simulink library "courseFollow_cl"  (R2018b)
settings: Solver=VariableStepAuto  StartTime=0.0  StopTime=10.0  RelTol=1e-3
undefined symbols (not defined in the file or in its folder): a
libraries: schmehlTangentRotation_ul x1, angleBtw2DVecs_ul x1
settings Model: Creator=James Reed  LastModifiedBy=jldanie5

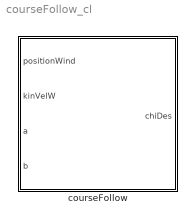
== system courseFollow_cl ==
  courseFollow : Subsystem

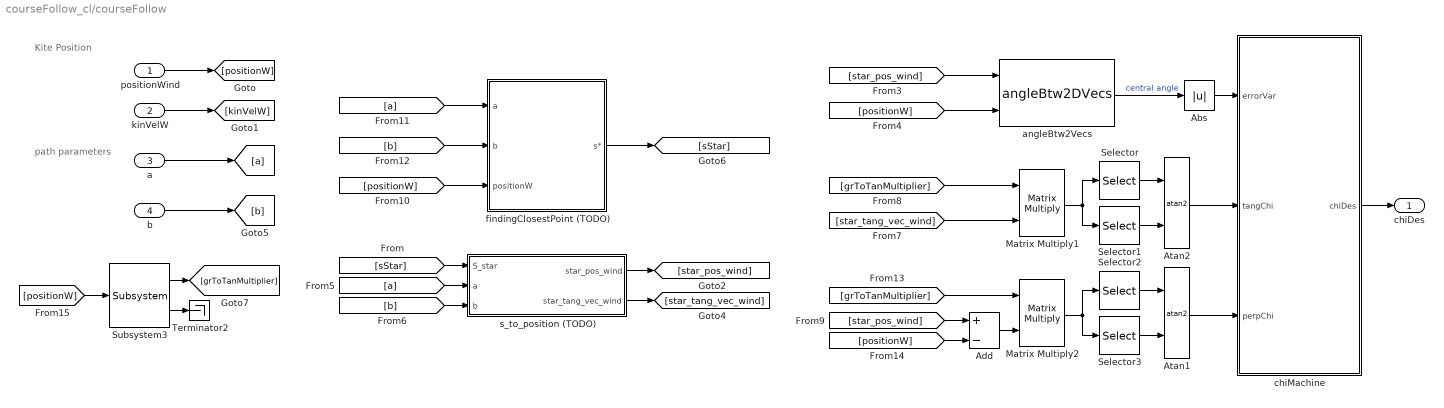
== system courseFollow_cl/courseFollow ==
  note: Kite Position
  note: path parameters
  "positionWind " : Inport
  kinVelW : Inport  Port=2
  a : Inport  Port=3
  "b " : Inport  Port=4
  Abs : Abs
  Add : Sum  Inputs=+-
  Atan1 : Trigonometry  Operator=atan2
  Atan2 : Trigonometry  Operator=atan2
  Matrix Multiply1 : Product  Multiplication=Matrix(*)
  Matrix Multiply2 : Product  Multiplication=Matrix(*)
  Selector : Selector  InputPortWidth=3  IndexOptions=Index vector (dialog)  Indices=2  OutputSizes=1
  Selector1 : Selector  InputPortWidth=3  IndexOptions=Index vector (dialog)  Indices=1  OutputSizes=1
  Selector2 : Selector  InputPortWidth=3  IndexOptions=Index vector (dialog)  Indices=2  OutputSizes=1
  Selector3 : Selector  InputPortWidth=3  IndexOptions=Index vector (dialog)  Indices=1  OutputSizes=1
  Subsystem3 : schmehlTangentRotation_ul/Subsystem  SystemSampleTime=-1
  Terminator2 : Terminator
  angleBtw2Vecs : angleBtw2DVecs_ul/angleBtw2DVecs  SystemSampleTime=-1
  chiMachine : Subsystem  mask{error_upper_lim=10*pi/180}
      mask prompts: error_upper_lim "Value of Error yielding 100% perpendicular"
  findingClosestPoint (TODO) : Subsystem
  s_to_position (TODO) : Subsystem
  "chiDes " : Outport
  wires:
  "positionWind "/1 -> [positionW]
  chiMachine/1("chiDes ") -> "chiDes "/1
  [positionW] -> findingClosestPoint (TODO)/3(positionW)
  a/1 -> [a]
  "b "/1 -> [b]
  [a] -> findingClosestPoint (TODO)/1(a)
  [b] -> findingClosestPoint (TODO)/2(b)
  findingClosestPoint (TODO)/1(s*) -> [sStar]
  [positionW] -> Subsystem3/1
  Subsystem3/2 -> Terminator2/1
  Subsystem3/1 -> [grToTanMultiplier]
  kinVelW/1 -> [kinVelW]
  [sStar] -> s_to_position (TODO)/1(S_star)
  s_to_position (TODO)/1(star_pos_wind) -> [star_pos_wind]
  [star_pos_wind] -> angleBtw2Vecs/1
  [positionW] -> angleBtw2Vecs/2
  angleBtw2Vecs/1 -> Abs/1  "central angle"
  Abs/1 -> chiMachine/1("errorVar ")
  [a] -> s_to_position (TODO)/2(a)
  [b] -> s_to_position (TODO)/3(b)
  s_to_position (TODO)/2(star_tang_vec_wind) -> [star_tang_vec_wind]
  Matrix Multiply1/1 -> Selector1/1, Selector/1
  [star_tang_vec_wind] -> Matrix Multiply1/2
  [grToTanMultiplier] -> Matrix Multiply1/1
  Selector/1 -> Atan2/1
  Selector1/1 -> Atan2/2
  Atan2/1 -> chiMachine/2(tangChi)
  [grToTanMultiplier] -> Matrix Multiply2/1
  Selector3/1 -> Atan1/2
  Matrix Multiply2/1 -> Selector3/1, Selector2/1
  Atan1/1 -> chiMachine/3("perpChi ")
  Selector2/1 -> Atan1/1
  Add/1 -> Matrix Multiply2/2
  [star_pos_wind] -> Add/1
  [positionW] -> Add/2

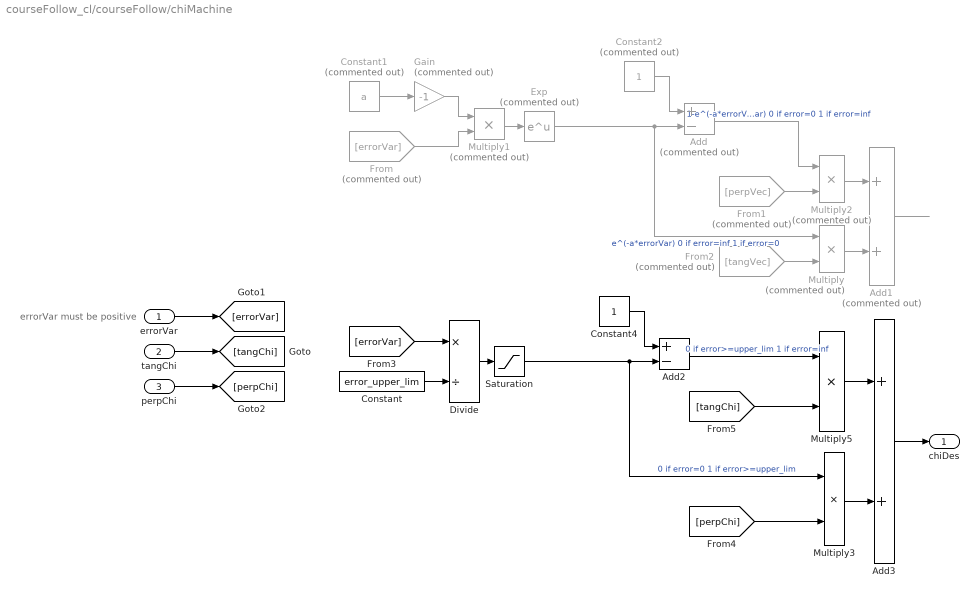
== system courseFollow_cl/courseFollow/chiMachine ==
  note: errorVar must be positive
  "errorVar " : Inport
  tangChi : Inport  Port=2
  "perpChi " : Inport  Port=3
  Add : Sum  Commented=on  Inputs=+-
  Add1 : Sum  Commented=on
  Add2 : Sum  Inputs=+-
  Add3 : Sum
  Constant : Constant  Value=error_upper_lim
  Constant1 : Constant  Commented=on  Value=a
  Constant2 : Constant  Commented=on
  Constant4 : Constant
  Divide : Product  Inputs=*/
  Exp : Math  Commented=on  SaturateOnIntegerOverflow=on
  From : From  Commented=on  GotoTag=errorVar
  From1 : From  Commented=on  GotoTag=perpVec
  From2 : From  Commented=on  GotoTag=tangVec
  Gain : Gain  Commented=on  Gain=-1
  Multiply : Product  Commented=on
  Multiply1 : Product  Commented=on
  Multiply2 : Product  Commented=on
  Multiply3 : Product
  Multiply5 : Product
  Saturation : Saturate  UpperLimit=1  LowerLimit=0
  "chiDes " : Outport
  wires:
  tangChi/1 -> [tangChi]
  Constant1/1 -> Gain/1
  Gain/1 -> Multiply1/1
  Multiply1/1 -> Exp/1
  Exp/1 -> Multiply/1, Add/2  "e^(-a*errorVar) 0 if error=inf 1 if error=0"
  Constant2/1 -> Add/1
  Add/1 -> Multiply2/1  "1-e^(-a*errorVar) 0 if error=0 1 if error=inf"
  Add1/1 -> ?
  "errorVar "/1 -> [errorVar]
  "perpChi "/1 -> [perpChi]
  From/1 -> Multiply1/2
  Multiply2/1 -> Add1/1
  Multiply/1 -> Add1/2
  From1/1 -> Multiply2/2
  From2/1 -> Multiply/2
  Constant4/1 -> Add2/1
  Saturation/1 -> Multiply3/1, Add2/2  "0 if error=0 1 if error>=upper_lim"
  Add3/1 -> "chiDes "/1
  Multiply3/1 -> Add3/2
  Multiply5/1 -> Add3/1
  Add2/1 -> Multiply5/1  "0 if error>=upper_lim 1 if error=inf"
  [errorVar] -> Divide/1
  Constant/1 -> Divide/2
  Divide/1 -> Saturation/1
  [tangChi] -> Multiply5/2
  [perpChi] -> Multiply3/2

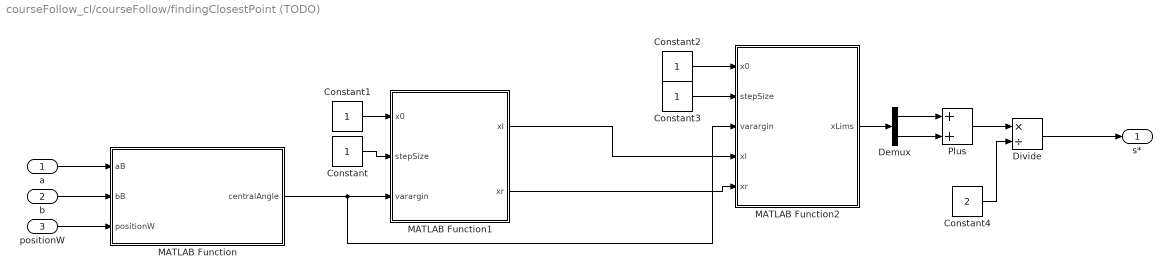
== system courseFollow_cl/courseFollow/findingClosestPoint (TODO) ==
  a : Inport
  b : Inport  Port=2
  positionW : Inport  Port=3
  Constant{,1..3} (4 alike) : Constant
  Constant4 : Constant  Value=2
  Demux : Demux  Outputs=2
  Divide : Product  Inputs=*/
  MATLAB Function : MATLAB Function  TreatAsAtomicUnit=on
  MATLAB Function1 : MATLAB Function  TreatAsAtomicUnit=on
  MATLAB Function2 : MATLAB Function  TreatAsAtomicUnit=on
  Plus : Sum
  s* : Outport
  wires:
  Constant2/1 -> MATLAB Function2/1(x0)
  Constant3/1 -> MATLAB Function2/2(stepSize)
  Constant1/1 -> MATLAB Function1/1(x0)
  Constant/1 -> MATLAB Function1/2(stepSize)
  MATLAB Function/1(centralAngle) -> MATLAB Function2/3(varargin), MATLAB Function1/3(varargin)
  MATLAB Function1/1(xl) -> MATLAB Function2/4(xl)
  MATLAB Function1/2(xr) -> MATLAB Function2/5(xr)
  MATLAB Function2/1(xLims) -> Demux/1
  Demux/2 -> Plus/2
  Demux/1 -> Plus/1
  Plus/1 -> Divide/1
  Constant4/1 -> Divide/2
  Divide/1 -> s*/1
  a/1 -> MATLAB Function/1(aB)
  b/1 -> MATLAB Function/2(bB)
  positionW/1 -> MATLAB Function/3(positionW)

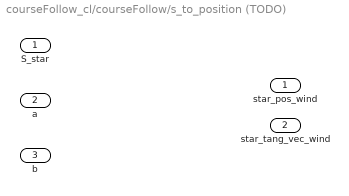
== system courseFollow_cl/courseFollow/s_to_position (TODO) ==
  S_star : Inport
  a : Inport  Port=2
  b : Inport  Port=3
  star_pos_wind : Outport
  star_tang_vec_wind : Outport  Port=2

== matlab function courseFollow_cl/courseFollow/findingClosestPoint (TODO)/MATLAB Function ==
  data: aB input; centralAngle output; bB input; positionW input
function centralAngle  = fcn(aB,bB,positionW)

lambda_g = (aB.*sin(s))./(1 + ((aB/bB)^2).*(cos(s).^2)); %path longitude
phi_g  = (10*pi/180)+(((aB/bB)^2).*sin(s).*cos(s))./(1 + ((aB/bB)^2).*(cos(s).^2)); %path latitude

path = [ cos(lambda_g).*cos(phi_g);
         sin(lambda_g).*cos(phi_g);
         sin(phi_g);]; 
      pathFunction = @(s) path ;
     centralAngle = @(s)2*asin(.5*(norm(pathFunction(s)-currentPosition)));

== matlab function courseFollow_cl/courseFollow/findingClosestPoint (TODO)/MATLAB Function1 ==
  data: x0 input; xl output; stepSize input; varargin input; xr output
function [xl,xr] = bound(x0, stepSize,varargin)

p = inputParser;

% Number of iterations before stopping attempt to tune step size
addOptional(p,'StepTimeout',1000,@(x) isnumeric(x) && isscalar(x))
% How much to increase the step size at every iteration
addOptional(p,'StepSizeMultiplier',2,@(x) isnumeric(x) && isscalar(x)  && x>=1)
% Number of iterations before quitting bounding phase
addOptional(p,'BoundingTimeout',1000,@(x) isnumeric(x) && isscalar(x))
% Handle of the function that you want to minimize
addOptional(p,'FunctionHandle',@objF,@(x) isa(x,'function_handle'))
% Initial point/guess
addRequired(p,'x0',@(x) isnumeric(x) && isvector(x))
% Step size
addRequired(p,'StepSize',@(x) isnumeric(x) && isscalar(x) && x>0)

parse(p,x0,stepSize,varargin{:})

fHandle  = p.Results.FunctionHandle;
stepSize = p.Results.StepSize;
x0       = p.Results.x0;

for tryCount = 1:p.Results.StepTimeout
    if fHandle(x0-stepSize) >= fHandle(x0) &&...
            fHandle(x0) >= fHandle(x0+stepSize)
        sign = +1;
        break
    elseif  fHandle(x0-stepSize) <= fHandle(x0) &&...
            fHandle(x0) <= fHandle(x0+stepSize)
        sign = -1;
        break
    end
    stepSize = stepSize/2^tryCount;
end

xCurrent = x0;
for ii = 0:p.Results.BoundingTimeout-1
    xRight = xCurrent + sign*stepSize*p.Results.StepSizeMultiplier^ii;
    if fHandle(xRight)>fHandle(xCurrent)
        break
    end
    xLeft = xCurrent;
    xCurrent = xRight;
end

if sign == -1
   xTemp  = sort([xLeft xRight]) ;
   xl  = xTemp(1);
   xr = xTemp(2);
end

end

== matlab function courseFollow_cl/courseFollow/findingClosestPoint (TODO)/MATLAB Function2 ==
  data: x0 input; xLims output; stepSize input; varargin input; xl input; xr input
function xLims = goldenSection(x0,stepSize,varargin,xl,xr)
% Function to implement golden section to minimize a scalar function
%
% Required Inputs
% x0       - initial guess
% stepSize - initial step size (step size may be reduced if this is too
% big)
%
% Optional Inputs
% DisplayOutput -  true/false prints output to command window
% MaxIterations - Maximum number of iterations before quitting, default =
% 1000
% FunctionConvergence - convergence criteria for function value, set to
% zero to disable, default = 0.01
% InputConvergence - convergence criteria for function input, set to zero
% to disable, default = 0.01
% StepTimeout - Max number of iterations for bounding phase step size
% reduction, default = 1000
% BoundingTimeout - Max number of iterations for bounding phase, default =
% 1000
 

% Input parsing
p = inputParser;
addRequired(p,'x0',@(x) isnumeric(x) && isscalar(x))
addRequired(p,'StepSize',@(x) isnumeric(x) && isscalar(x) && x>0)
addOptional(p,'DisplayOutput',false,@(x) islogical(x))
addOptional(p,'MaxIterations',1000,@(x) isnumeric(x) && isscalar(x) && x>0)
addOptional(p,'FunctionConvergence',0.00001,@(x) isnumeric(x) && isscalar(x) && x>=0)
addOptional(p,'InputConvergence',0.0001,@(x) isnumeric(x) && isscalar(x) && x>=0)
addOptional(p,'StepTimeout',1000,@(x) isnumeric(x) && isscalar(x))
addOptional(p,'StepSizeMultiplier',2,@(x) isnumeric(x) && isscalar(x)  && x>=1)
addOptional(p,'BoundingTimeout',1000,@(x) isnumeric(x) && isscalar(x))
addOptional(p,'FunctionHandle',@objF,@(x) isa(x,'function_handle'))
parse(p,x0,stepSize,varargin{:})

% Rename some variables to clean up code later on
fHandle  = p.Results.FunctionHandle;
stepSize = p.Results.StepSize;
x0       = p.Results.x0;

% Bounding Phase
[xl,xr] = bound(x0,stepSize,'FunctionHandle',p.Results.FunctionHandle,...
    'StepTimeout',p.Results.StepTimeout,...
    'StepSizeMultiplier',p.Results.StepSizeMultiplier,...
    'BoundingTimeout',p.Results.BoundingTimeout,...
    'FunctionHandle',p.Results.FunctionHandle);

% Begin golden section
tau = 1 - 0.38197;
initialRange = abs(xr-xl);
fl = fHandle(xl);
fr = fHandle(xr);
% Print column headers to command window for output
if p.Results.DisplayOutput
    headings = {'xl','Fl','x1','F1','x2','F2','xr','Fr','xOpt','FOpt'};
    headingString = [' '];
    for ii = 1:length(headings)
        headingString = [headingString pad(headings{ii},11)];
    end
    fprintf(['\n' headingString '\n'])
end

for ii = 1:p.Results.MaxIterations
    xTwo = (1-tau)*xl+tau*xr;
    xOne = tau*xl+(1-tau)*xr;
    fOne = fHandle(xOne);
    fTwo = fHandle(xTwo);
    fMin = min([fl fr fOne fTwo]);
    fMax = max([fl fr fOne fTwo]);
    xMin = min([xl xr xOne xTwo]);
    xMax = max([xl xr xOne xTwo]);
    if abs((fMax-fMin)/fMin)<= p.Results.FunctionConvergence || ...
            abs((xMax - xMin)/initialRange) <= p.Results.InputConvergence
        if p.Results.DisplayOutput
            fprintf('\nSolution converged.  Stopping program.\n')
        end
        break
    end
    if fOne>fTwo
        xl = xOne;
        f1 = fOne;
    else
        xr = xTwo;
        fr = fTwo;
    end
end

% xTest = linspace(-1,1,1000);
% for ii = 1:length(xTest)
%     y(ii) = fHandle(xTest(ii));
% end
% plot(xTest,y)

xLims = [xl xr];
end
